simulink model "MCASSimulation"  (R2022b)
settings: Solver=VariableStepAuto  StartTime=0.0  StopTime=120  RelTol=1e-3
model workspace (MAT data in the model file):
  ASd = 1
values from neighbouring files (symbols this model uses):
  sortedParams = table2struct(sortedT)    [RunSimulations.m]    (also in no_anomolies_run_handler.m)
libraries: slpidlib x12, simulink_extras x3
(part 4 of 4)

== matlab function MCASSimulation/Human Pilot Simulator/Throttle Controller/MATLAB Function ==
  data: mode input; s1 output; s2 output
% "0" puts a switch in the "down" position.

function [s1, s2] = mode_selector(mode)

switch mode
    case 0  % off
        s1 = 1;
        s2 = 1;
    case 1  % airspeed
        s1 = 0;
        s2 = 0;
    case 2  % direct
        s1 = 0;
        s2 = 1;
    otherwise
        error("throttle mode invalid");

end

== matlab function MCASSimulation/Human Pilot Simulator/Aileron Controller/MATLAB Function1 ==
  data: mode input; s1 output; s2 output; s3 output
% "0" puts a switch in the "down" position.

function [s1, s2, s3]  = mode_selector(mode)

switch mode
    case 0  % off
        s1 = 1;
        s2 = 1;
        s3 = 1;
    case 1  % heading
        s1 = 0;
        s2 = 0;
        s3 = 0;
    case 2 % heading rate
        s1 = 0;
        s2 = 0;
        s3 = 1;
    case 3 % roll angle
        s1 = 0;
        s2 = 1;
        s3 = 1;
    otherwise
        error("aileron mode invalid");

end

== matlab function MCASSimulation/Human Pilot Simulator/Rudder Controller/MATLAB Function1 ==
  data: mode input; s1 output
% "0" puts a switch in the "down" position.

function s1 = mode_selector(mode)

switch mode
    case 0  % off
        s1 = 1;
    case 1  % minimize sideslip (beta)
        s1 = 0;
    otherwise
        error("rudder mode invalid");

end
